simulink model "threephase_SVPWM"  (R2015a)
settings: Solver=ode45  StartTime=0.0  StopTime=0.2  MaxStep=0.00001  MinStep=0.000001  RelTol=1e-3
libraries: powerlib x10, powerlib_meascontrol x3, simulink x1
settings Model: Creator=hp  LastModifiedBy=hp
settings SolverCC: ZeroCrossControl=DisableAll

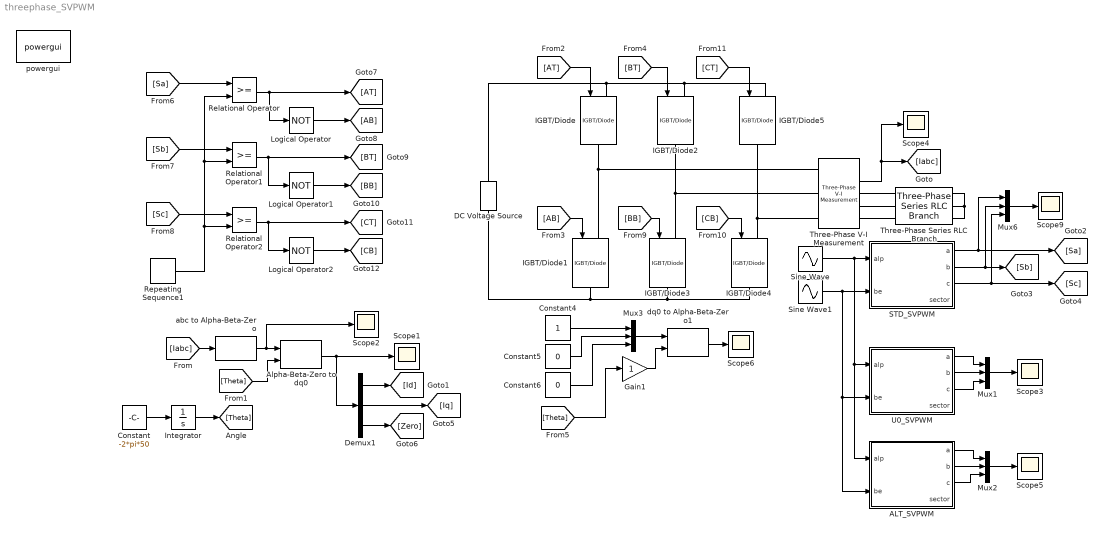
== system threephase_SVPWM ==
  ALT_SVPWM : MATLAB Function  TreatAsAtomicUnit=on
  Alpha-Beta-Zero to dq0 : powerlib_meascontrol/Transformations/Alpha-Beta-Zero to dq0  Alignment=Aligned with phase A axis
  Constant : Constant  Value=-2*pi*50
  Constant4 : Constant
  Constant5 : Constant  Value=0
  Constant6 : Constant  Value=0
  DC Voltage Source : powerlib/Electrical Sources/DC Voltage Source  Amplitude=400  Measurements=None
  Demux1 : Demux  Outputs=3
  Gain1 : Gain
  IGBT/Diode{,1..5} (6 alike) : powerlib/Power Electronics/IGBT//Diode  Ron=1e-3  Rs=1e5  Cs=inf  Measurements=off
  Integrator : Integrator
  Logical Operator : Logic  Operator=NOT  Inputs=1  AllPortsSameDT=off  OutDataTypeStr=boolean
  Logical Operator1 : Logic  Operator=NOT  Inputs=1  AllPortsSameDT=off  OutDataTypeStr=boolean
  Logical Operator2 : Logic  Operator=NOT  Inputs=1  AllPortsSameDT=off  OutDataTypeStr=boolean
  Mux{1..3,6} (4 alike) : Mux  Inputs=3
  Relational Operator : RelationalOperator  OutDataTypeStr=boolean
  Relational Operator1 : RelationalOperator  OutDataTypeStr=boolean
  Relational Operator2 : RelationalOperator  OutDataTypeStr=boolean
  Repeating Sequence1 : simulink/Sources/Repeating Sequence  rep_seq_t=[0 0.5 1]/1000  rep_seq_y=[0 1 0]
  STD_SVPWM : MATLAB Function  TreatAsAtomicUnit=on
  Scope{1..6,9} (7 alike) : Scope
      Scope1 settings: YMin=-22.5  YMax=7.5
      Scope2 settings: YMin=-25  YMax=25  SaveName=ScopeData2
      Scope3 settings: YMin=0  YMax=1
      Scope4 settings: YMin=-25  YMax=25  SaveName=ScopeData5
      Scope5 settings: YMin=0  YMax=1  SaveName=ScopeData3
      Scope6 settings: YMin=-1  YMax=1  SaveName=ScopeData6
      Scope9 settings: YMin=0  YMax=1  SaveName=ScopeData8
  Sine Wave : Sin  Frequency=2*pi*50  SampleTime=0
  Sine Wave1 : Sin  Frequency=2*pi*50  Phase=pi/2  SampleTime=0
  Three-Phase Series RLC Branch : powerlib/Elements/Three-Phase Series RLC Branch  LConnTagsString=A|B|C  RConnTagsString=A|B|C  BranchType=RLC  Resistance=10  Inductance=10e-3  Capacitance=0  Measurements=None
  Three-Phase V-I Measurement : powerlib/Measurements/Three-Phase V-I Measurement  VoltageMeasurement=phase-to-phase  SetLabelV=off  LabelV=Vabc  Vpu=off  VpuLL=off  CurrentMeasurement=yes  SetLabelI=off  LabelI=Iabc  Ipu=off  Pbase=100e6  Vbase=500e3  OutputType=Complex  PhasorSimulation=off  PSBequivalent=0
  U0_SVPWM : MATLAB Function  TreatAsAtomicUnit=on
  abc to Alpha-Beta-Zero : powerlib_meascontrol/Transformations/abc to Alpha-Beta-Zero
  dq0 to Alpha-Beta-Zero1 : powerlib_meascontrol/Transformations/dq0 to Alpha-Beta-Zero  Alignment=Aligned with phase A axis
  powergui : powerlib/powergui  Priority=1  SimulationMode=Continuous  SolverType=Tustin/Backward Euler (TBE)  SampleTime=2e-6  frequency=60  SPID=off  DisableSnubberDevices=off  DisableRonSwitches=off  DisableVfSwitches=off  SwTol=0  DisplayEquations=off  Interpol=off  methode=off  Ts=100  FunctionMessages=off  echomessages=off  HookPort=off  EnableUseOfTLC=off  x0status=blocks  frequencyindice=0  Pbase=100e6  ErrMax=1e-4  Iterations=50  UnitsV=kV  UnitsW=MW  buscounter=0  RestoreLinks=warning  ResistiveCurrentMeasurement=off  Frange=[0:2:500]  Ylog=off  Xlog=on  ShowGrid=off  save=off  variable=ZData  structure=0  ZoomFFT=off  StartTime=0.0  cycles=1  DisplayStyle=1  fundamental=60  FreqAxis=off  MaxFrequency=1000  frequencyindicesteady=1  RmsSteady=1  display=off
  wires:
  Three-Phase V-I Measurement/2 -> Scope4/1, [Iabc]
  [Iabc] -> abc to Alpha-Beta-Zero/1
  Alpha-Beta-Zero to dq0/1 -> Demux1/1, Scope1/1
  Constant/1 -> Integrator/1
  abc to Alpha-Beta-Zero/1 -> Scope2/1, Alpha-Beta-Zero to dq0/1
  Integrator/1 -> [Theta]
  [Theta] -> Alpha-Beta-Zero to dq0/2
  Demux1/1 -> [Id]
  Demux1/2 -> [Iq]
  Demux1/3 -> [Zero]
  dq0 to Alpha-Beta-Zero1/1 -> Scope6/1
  Mux3/1 -> dq0 to Alpha-Beta-Zero1/1
  Gain1/1 -> dq0 to Alpha-Beta-Zero1/2
  Constant4/1 -> Mux3/1
  Constant6/1 -> Mux3/3
  Constant5/1 -> Mux3/2
  [Theta] -> Gain1/1
  [Sa] -> Relational Operator/1
  Repeating Sequence1/1 -> Relational Operator2/2, Relational Operator/2, Relational Operator1/2
  [Sb] -> Relational Operator1/1
  [Sc] -> Relational Operator2/1
  Relational Operator/1 -> Logical Operator/1, [AT]
  Logical Operator/1 -> [AB]
  Relational Operator1/1 -> Logical Operator1/1, [BT]
  Logical Operator1/1 -> [BB]
  Relational Operator2/1 -> Logical Operator2/1, [CT]
  Logical Operator2/1 -> [CB]
  [AT] -> IGBT/Diode/1
  [AB] -> IGBT/Diode1/1
  [BT] -> IGBT/Diode2/1
  [BB] -> IGBT/Diode3/1
  [CB] -> IGBT/Diode4/1
  [CT] -> IGBT/Diode5/1
  STD_SVPWM/1(a) -> Mux6/1, [Sa]
  STD_SVPWM/2(b) -> Mux6/2, [Sb]
  STD_SVPWM/3(c) -> Mux6/3, [Sc]
  Mux6/1 -> Scope9/1
  U0_SVPWM/1(a) -> Mux1/1
  U0_SVPWM/2(b) -> Mux1/2
  U0_SVPWM/3(c) -> Mux1/3
  Mux1/1 -> Scope3/1
  Sine Wave/1 -> ALT_SVPWM/1(alp), U0_SVPWM/1(alp), STD_SVPWM/1(alp)
  Sine Wave1/1 -> ALT_SVPWM/2(be), U0_SVPWM/2(be), STD_SVPWM/2(be)
  Mux2/1 -> Scope5/1
  ALT_SVPWM/1(a) -> Mux2/1
  ALT_SVPWM/2(b) -> Mux2/2
  ALT_SVPWM/3(c) -> Mux2/3
  connections:
  Three-Phase Series RLC Branch/RConn1 -- Three-Phase Series RLC Branch/RConn2 -- Three-Phase Series RLC Branch/RConn3
  Three-Phase V-I Measurement/RConn1 -- Three-Phase Series RLC Branch/LConn1
  Three-Phase V-I Measurement/RConn2 -- Three-Phase Series RLC Branch/LConn2
  Three-Phase V-I Measurement/RConn3 -- Three-Phase Series RLC Branch/LConn3
  IGBT/Diode/RConn1 -- IGBT/Diode1/LConn1 -- Three-Phase V-I Measurement/LConn1
  IGBT/Diode2/RConn1 -- Three-Phase V-I Measurement/LConn2 -- IGBT/Diode3/LConn1
  IGBT/Diode5/RConn1 -- Three-Phase V-I Measurement/LConn3 -- IGBT/Diode4/LConn1
  IGBT/Diode1/RConn1 -- DC Voltage Source/LConn1 -- IGBT/Diode3/RConn1 -- IGBT/Diode4/RConn1
  IGBT/Diode/LConn1 -- IGBT/Diode2/LConn1 -- IGBT/Diode5/LConn1 -- DC Voltage Source/RConn1

== matlab function threephase_SVPWM/U0_SVPWM ==
  data: alp input; a output; be input; b output; c output; sector output
function [a,b,c,sector] = fcn(alp,be)
%#codegen
	sec_a=0,sec_b=0,sec_c=0;
	t_o = 0,ta = 0,tb = 0,tc = 0,tsec = 0;

    sec_a = be;										%Beta;
	sec_b = ((-be/2)+(alp*0.866));			%(-0.5*Beta+(0.866*alpha));
	sec_c = ((-be/2)-(alp*0.866));			%(-0.5*Beta-(0.866*alpha));
    
    if(sec_a>=0)
       if(sec_b>=0)
       												%	sector 1
    								%	t_1 = sec_b, t_2 =sec_a
    		ta = sec_a+sec_b;
    		tb  = sec_a;
    		tc  = 0;
            tsec = 1;
       else
            if(sec_c>=0)												%	sector 3
        								%	t_1 = sec_a, t_2 =sec_c
        		ta = 0;
        		tb = sec_a+sec_c;
        		tc = sec_c;
                tsec = 3;
            else												%	sector 2
        							%	t_1 = -sec_c, t_2 =-sec_b
        		ta = -sec_c;
        		tb = -(sec_c+sec_b);
        		tc = 0;
                tsec = 2;
            end
       end
    else
       if(sec_b>=0)
           if(sec_c>=0)                                                  %	sector 5
        						%	t_1 = sec_c, t_2 =sec_b
        		ta = sec_b;
        		tb = 0;
        		tc = sec_c+sec_b;
                tsec = 5;
           else                                                  %	sector 6
        	 				%	t_1 = -sec_a, t_2 =-sec_c
        		ta = -(sec_a+sec_c);
        		tb = 0;
        		tc = -sec_a;
                tsec = 6;
           end
       else
            if(sec_c>=0)                                      %	sector 4
        					%	t_1 = -sec_b, t_2 =-sec_a
        		ta = 0;
        		tb = -sec_b;
        		tc = -(sec_a+sec_b);
                tsec = 4;
            end
       end
    end
a = ta;
b = tb;
c = tc;
sector = tsec;

== matlab function threephase_SVPWM/STD_SVPWM ==
  data: alp input; a output; be input; b output; c output; sector output
function [a,b,c,sector] = fcn(alp,be)
%#codegen
	sec_a=0,sec_b=0,sec_c=0;
	t_o = 0,ta = 0,tb = 0,tc = 0,tsec = 0;

    sec_a = be;										%Beta;
	sec_b = ((-be/2)+(alp*0.866));			%(-0.5*Beta+(0.866*alpha));
	sec_c = ((-be/2)-(alp*0.866));			%(-0.5*Beta-(0.866*alpha));
    
    if(sec_a>=0)
       if(sec_b>=0)
       												%	sector 1
    		t_o = (1 - (sec_a+sec_b))/2;							%	t_1 = sec_b, t_2 =sec_a
    		ta = sec_a+sec_b+(t_o);
    		tb  = sec_a+(t_o);
    		tc  = (t_o);
            tsec = 1;
       else
            if(sec_c>=0)												%	sector 3
        		t_o = (1 - (sec_a+sec_c))/2;						%	t_1 = sec_a, t_2 =sec_c
        		ta = (t_o);
        		tb = sec_a+sec_c+(t_o);
        		tc = sec_c+(t_o);
                tsec = 3;
            else												%	sector 2
        		t_o = (1 + (sec_c+sec_b))/2;					%	t_1 = -sec_c, t_2 =-sec_b
        		ta = -sec_c+(t_o);
        		tb = -(sec_c+sec_b)+(t_o);
        		tc = (t_o);
                tsec = 2;
            end
       end
    else
       if(sec_b>=0)
           if(sec_c>=0)                                                  %	sector 5
        		t_o = (1 - (sec_c+sec_b))/2; 				%	t_1 = sec_c, t_2 =sec_b
        		ta = sec_b+(t_o);
        		tb = (t_o);
        		tc = sec_c+sec_b+(t_o);
                tsec = 5;
           else                                                  %	sector 6
        		t_o = (1 + (sec_a+sec_c))/2; 				%	t_1 = -sec_a, t_2 =-sec_c
        		ta = -(sec_a+sec_c)+(t_o);
        		tb = (t_o);
        		tc = -sec_a+(t_o);
                tsec = 6;
           end
       else
            if(sec_c>=0)                                      %	sector 4
        		t_o = (1 + (sec_a+sec_b))/2;			%	t_1 = -sec_b, t_2 =-sec_a
        		ta = (t_o);
        		tb = -sec_b+(t_o);
        		tc = -(sec_a+sec_b)+(t_o);
                tsec = 4;
            end
       end
    end
a = ta;
b = tb;
c = tc;
sector = tsec;

== matlab function threephase_SVPWM/ALT_SVPWM ==
  data: alp input; a output; be input; b output; c output; sector output
function [a,b,c,sector] = fcn(alp,be)
%#codegen
	sec_a=0,sec_b=0,sec_c=0;
	t_o = 0,ta = 0,tb = 0,tc = 0,tsec = 0;

    sec_a = be;										%Beta;
	sec_b = ((-be/2)+(alp*0.866));			%(-0.5*Beta+(0.866*alpha));
	sec_c = ((-be/2)-(alp*0.866));			%(-0.5*Beta-(0.866*alpha));
    
    if(sec_a>=0)
       if(sec_b>=0)
       												%	sector 1
    		t_o = (1 - (sec_a+sec_b))/2;							%	t_1 = sec_b, t_2 =sec_a
    		ta = 1;
    		tb  = sec_a+(t_o);
    		tc  = (t_o);
            tsec = 1;
       else
            if(sec_c>=0)												%	sector 3
        		t_o = (1 - (sec_a+sec_c))/2;						%	t_1 = sec_a, t_2 =sec_c
        		ta = (t_o);
        		tb = 1;
        		tc = sec_c+(t_o);
                tsec = 3;
            else												%	sector 2
        		t_o = (1 + (sec_c+sec_b))/2;					%	t_1 = -sec_c, t_2 =-sec_b
        		ta = -sec_c;
        		tb = -(sec_c+sec_b);
        		tc = 0;
                tsec = 2;
            end
       end
    else
       if(sec_b>=0)
           if(sec_c>=0)                                                  %	sector 5
        		t_o = (1 - (sec_c+sec_b))/2; 				%	t_1 = sec_c, t_2 =sec_b
        		ta = sec_b+(t_o);
        		tb = (t_o);
        		tc = 1;
                tsec = 5;
           else                                                  %	sector 6
        		t_o = (1 + (sec_a+sec_c))/2; 				%	t_1 = -sec_a, t_2 =-sec_c
        		ta = -(sec_a+sec_c);
        		tb = 0;
        		tc = -sec_a;
                tsec = 6;
           end
       else
            if(sec_c>=0)                                      %	sector 4
        		t_o = (1 + (sec_a+sec_b))/2;			%	t_1 = -sec_b, t_2 =-sec_a
        		ta = 0;
        		tb = -sec_b;
        		tc = -(sec_a+sec_b);
                tsec = 4;
            end
       end
    end
a = ta;
b = tb;
c = tc;
sector = tsec;
